simulink model "controller"  (Simulink 8.8)
settings: Solver=FixedStepDiscrete  StartTime=0.0  StopTime=CONFIG.TEnd  FixedStep=CONFIG.TS  RelTol=1e-3  EnableMultiTasking=on
InitFcn:
  | clc
  | cd(fileparts(which(bdroot)));
  | initTrqBalancingSeeSaw;
undefined symbols (not defined in the file): bVectorConstraints, CONFIG, Config, ConstraintsMatrix, directionOfOscillation, FRAMES, gain, LEFT_RIGHT_FOOT_IN_CONTACT, noOscillationTime, referenceParams, reg, ROBOT_DOF, sat, seesaw
libraries: WBToolboxLibrary x47
(part 2 of 2)

== matlab function Balancing controller and QP solver/  integral of H_r /MATLAB Function ==
  data: qjErr input double; JL input double; JR input double; vbEquivalent output double; reg parameter double; activeFeetConstraints input double
function vbEquivalent = generateReferencesForH(qjErr,JL,JR,reg,activeFeetConstraints)

% The approximation of integral of angular momentum is given by:
%
%    H_approx = JG(qRef)*(qj-qjDes)
%
% It is assumed here that one of the feet is always on ground at time t=0
% 
if activeFeetConstraints(1) == 1
    
    pinvJb             = (transpose(JL(:,1:6))*JL(:,1:6) + reg.pinvTolVb*eye(6))\transpose(JL(:,1:6));
    vbEquivalent       = -pinvJb*JL(:,7:end)*qjErr;
else
    
    pinvJb             = (transpose(JR(:,1:6))*JR(:,1:6) + reg.pinvTolVb*eye(6))\transpose(JR(:,1:6));
    vbEquivalent       = -pinvJb*JR(:,7:end)*qjErr;
end
end
